simulink model "RSC_RRT_Open_Loop"  (Simulink 7.6)
settings: Solver=ode3  StartTime=0.0  StopTime=10  FixedStep=.05  RelTol=1e-3
PostLoadFcn:
  | % Setup Segmentation parameters and java class
  | % For data parsing
  | 
  | % Distance away from car to be considered
  | Threshold = 15;
  | 
  | % Maximum number of points in a clustered object
  | MaxCluster = 25;
  | 
  | % Number of data points in Lidar array
  | % DO NOT CHANGE!
  | Num_Beams = 726;
  | Scaling = 1;
  | 
  | % Get current path and import Java class
  | javaaddpath({'/'});
  | import ClusterMethodNew.*;
  | 
  | % Define instance of the class
  | DataCluster = ClusterMethodNew(Threshold,MaxCluster,Scaling);
  | 
  | % Allow reading from the workspace
  | eml.extrinsic('evalin');
InitFcn:
  | % Setup MPC parameters and Global Variables
  | a2g = 1/9.81;
  | r2d = 180/pi;
  | K_sr = 15.97;
  | neutral_steer = 104;
  | s2t = (pi/180)*(1/K_sr);
  | 
  | A_kt =[         0         0         0         0         0         0
  |          0   -3.5058   -1.6990  -25.6114   -2.2435         0
  |          0    2.2782   -4.2575  -64.1772   -5.6218         0
  |          0         0    1.0000         0         0         0
  |          0   -0.0158    0.0295    0.4442   -4.1900         0
  |          0         0         0         0    1.0000         0];
  | 
  | 
  | B_kt =[0
  |    23.7845
  |   -16.0342
  |          0
  |    17.5770
  |          0];
  | 
  | load MPC_test_2
StartFcn:
  | % Initalize serial connection with LiDAR
StopFcn:
  | % Turn off Laser and Disconnect
undefined symbols (not defined in the file or in its folder): CR, serial
libraries: instrumentlib x3, mpclib x1, realtime_pacer_lib x1
settings Model: Creator=TCA  LastModifiedBy=ipainter  BufferReuse=off
settings OptimizationCC: BlockReduction=off  InlineParams=on  BufferReuse=off  InitFltsAndDblsToZero=on
settings DebuggingCC: AlgebraicLoopMsg=none  SolverPrmCheckMsg=none  UnconnectedInputMsg=none  UnconnectedOutputMsg=none  UnconnectedLineMsg=none  StrictBusMsg=Warning
settings SFSimCC: SimParseCustomCode=off

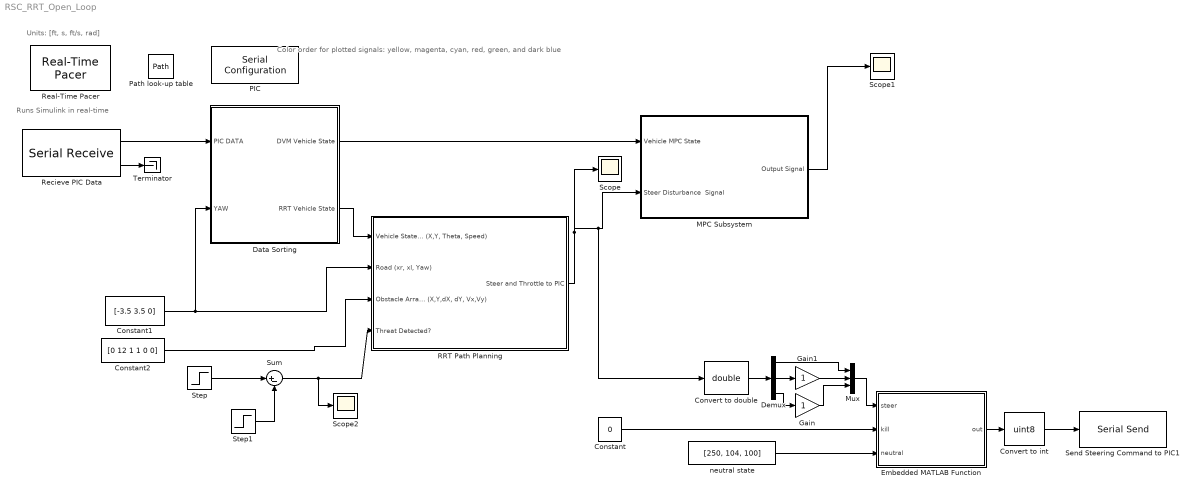
== system RSC_RRT_Open_Loop ==
  note: Runs Simulink
      |  in real-time
  note: Units: [ft, s, ft/s, rad]
  note: Color order for plotted signals:
      | yellow, magenta, cyan, red, green, and dark blue
  Constant : Constant  Value=0
  Constant1 : Constant  Value=[-3.5 3.5 0]
  Constant2 : Constant  Value=[0 12 1 1 0 0]
  Convert to double : DataTypeConversion  OutDataTypeStr=double  SampleTime=0.05  SaturateOnIntegerOverflow=on  RndMeth=Zero
  Convert to int : DataTypeConversion  OutDataTypeStr=uint8  SampleTime=0.05  SaturateOnIntegerOverflow=on  RndMeth=Zero
  Data Sorting : Subsystem
  Demux : Demux  Outputs=3
  Embedded MATLAB Function : Stateflow chart  TreatAsAtomicUnit=on
  Gain : Gain
  Gain1 : Gain
  MPC Subsystem : Subsystem
  Mux : Mux  Inputs=3
  PIC : instrumentlib/Serial Configuration  Priority=-200000  DialogController=instrumentcreatedialog  DialogControllerArgs=DataTag0  ComPortMenu=COM5  ComPort=COM5  ObjConstructor=serial('COM5');  BaudRate=9600  DataBits=8  Parity=none  StopBits=1  FlowControl=none  Timeout=10  ByteOrder=LittleEndian
  Path look-up table : DataStoreMemory  DataStoreName=Path  ReadBeforeWriteMsg=warning  WriteAfterWriteMsg=warning  WriteAfterReadMsg=warning  InitialValue=zeros(50, 6)  VectorParams1D=off
  RRT Path Planning : Subsystem
  Real-Time Pacer : realtime_pacer_lib/Real-Time Pacer  simTimePerRealTime=1
  Recieve PIC Data : instrumentlib/Serial Receive  DialogController=instrumentcreatedialog  DialogControllerArgs=DataTag1  ComPortMenu=COM5  ComPort=COM5  ObjConstructor=serial('COM5');  Terminator=CR ('\r')  DataSize="[1  16]"  DataType=uint8  EnableBlockingMode=off  ActionDataUnavailable=Output last received value  CustomValue=0  SampleTime=.05
  Scope : Scope
      settings: TimeRange=10  YMin=60  YMax=260
  Scope1 : Scope
  Scope2 : Scope
      settings: SaveName=ScopeData2
  Send Steering Command to PIC1 : instrumentlib/Serial Send  DialogController=instrumentcreatedialog  DialogControllerArgs=DataTag2  ComPortMenu=<Please select a port...>  ComPort=COM5  ObjConstructor=serial('COM5');  Header=250  Terminator=<none>  EnableBlockingMode=off
  Step : Step  Time=5  SampleTime=0
  Step1 : Step  Time=5.1  SampleTime=0
  Sum : Sum  Inputs=|+-
  Terminator : Terminator
  neutral state : Constant  Value=[250, 104, 100]
  wires:
  Data Sorting/2(RRT Vehicle State) -> RRT Path Planning/1("Vehicle State (X,Y, Theta, Speed)")
  neutral state/1 -> Embedded MATLAB Function/3(neutral)
  Embedded MATLAB Function/1(out) -> Convert to int/1
  Convert to double/1 -> Demux/1
  Demux/3 -> Gain/1
  Gain/1 -> Mux/3
  Demux/1 -> Mux/1
  Mux/1 -> Embedded MATLAB Function/1(steer)
  Demux/2 -> Gain1/1
  Gain1/1 -> Mux/2
  MPC Subsystem/1(Output Signal) -> Scope1/1
  Constant/1 -> Embedded MATLAB Function/2(kill)
  ? -> ?
  Recieve PIC Data/1 -> Data Sorting/1(PIC DATA)
  Recieve PIC Data/2 -> Terminator/1
  Constant2/1 -> RRT Path Planning/3("Obstacle Array (X,Y,dX, dY, Vx,Vy)")
  Constant1/1 -> RRT Path Planning/2("Road (xr, xl, Yaw)"), Data Sorting/2(" YAW")
  Data Sorting/1(DVM Vehicle State) -> MPC Subsystem/1(Vehicle MPC State)
  RRT Path Planning/1(Steer and Throttle to PIC) -> Scope/1, MPC Subsystem/2(Steer Disturbance  Signal), Convert to double/1
  Convert to int/1 -> Send Steering Command to PIC1/1
  Step/1 -> Sum/1
  Sum/1 -> RRT Path Planning/4(Threat Detected?), Scope2/1
  Step1/1 -> Sum/2

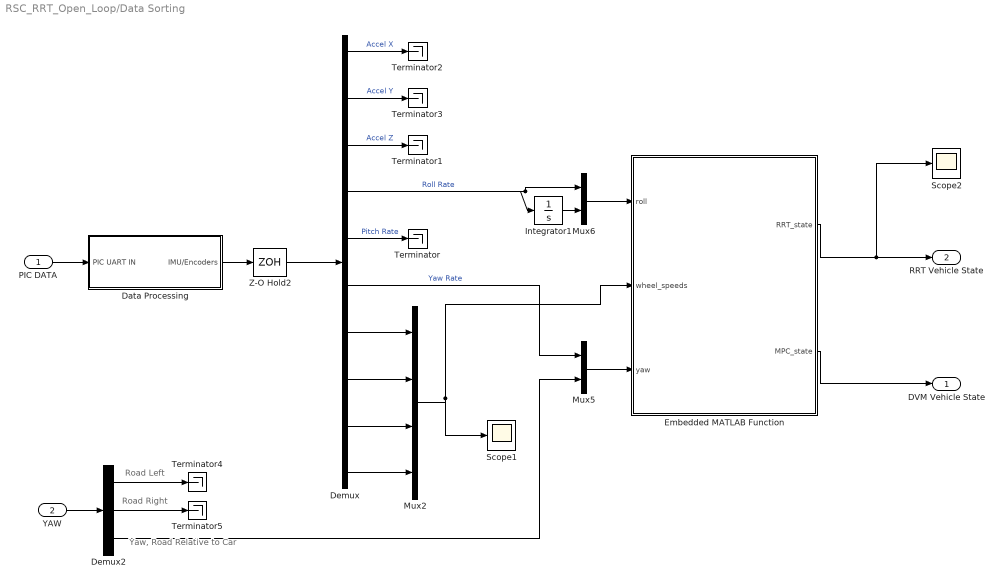
== system RSC_RRT_Open_Loop/Data Sorting ==
  note: Road Left
  note: Road Right
  note: Yaw, Road Relative to Car
  PIC DATA : Inport
  " YAW" : Inport  Port=2
  Data Processing : Subsystem
  Demux : Demux  Outputs=10
  Demux2 : Demux  Outputs=3
  Embedded MATLAB Function : Stateflow chart  TreatAsAtomicUnit=on
  Integrator1 : Integrator
  Mux2 : Mux
  Mux5 : Mux  Inputs=2
  Mux6 : Mux  Inputs=2
  Scope1 : Scope
      settings: SaveName=ScopeData3
  Scope2 : Scope
      settings: SaveName=ScopeData4
  Terminator{,1..5} (6 alike) : Terminator
  Z-O Hold2 : ZeroOrderHold  SampleTime=0.05
  DVM Vehicle State : Outport
  RRT Vehicle State : Outport  Port=2
  wires:
  Demux/6 -> Mux5/1  "Yaw Rate"
  Demux/2 -> Terminator3/1  "Accel Y"
  Demux/4 -> Mux6/1, Integrator1/1  "Roll Rate"
  Demux/5 -> Terminator/1  "Pitch Rate"
  Demux/7 -> Mux2/1
  Demux/8 -> Mux2/2
  Demux/9 -> Mux2/3
  Demux/10 -> Mux2/4
  Z-O Hold2/1 -> Demux/1
  Integrator1/1 -> Mux6/2
  Mux6/1 -> Embedded MATLAB Function/1(roll)
  Demux/1 -> Terminator2/1  "Accel X"
  Embedded MATLAB Function/2(MPC_state) -> DVM Vehicle State/1
  " YAW"/1 -> Demux2/1
  Demux/3 -> Terminator1/1  "Accel Z"
  Demux2/1 -> Terminator4/1
  Demux2/2 -> Terminator5/1
  Demux2/3 -> Mux5/2
  Mux5/1 -> Embedded MATLAB Function/3(yaw)
  Embedded MATLAB Function/1(RRT_state) -> RRT Vehicle State/1, Scope2/1
  Data Processing/1(IMU/Encoders) -> Z-O Hold2/1
  PIC DATA/1 -> Data Processing/1(PIC UART IN)
  Mux2/1 -> Embedded MATLAB Function/2(wheel_speeds), Scope1/1

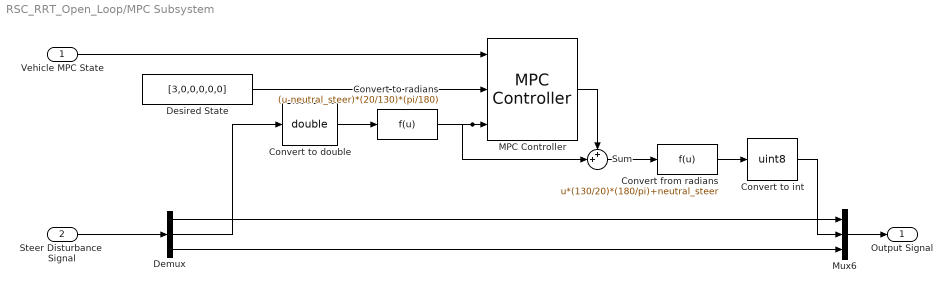
== system RSC_RRT_Open_Loop/MPC Subsystem ==
  Vehicle MPC State : Inport
  Steer Disturbance  Signal : Inport  Port=2
  Convert from radians : Fcn  Expr=u*(130/20)*(180/pi)+neutral_steer
  Convert to double : DataTypeConversion  OutDataTypeStr=double  SampleTime=.05  SaturateOnIntegerOverflow=on  RndMeth=Zero
  Convert to int : DataTypeConversion  OutDataTypeStr=uint8  SampleTime=.05  SaturateOnIntegerOverflow=on  RndMeth=Zero
  Convert to radians : Fcn  Expr=(u-neutral_steer)*(20/130)*(pi/180)
  Demux : Demux  Outputs=3
  Desired State : Constant  Value=[3,0,0,0,0,0]
  MPC Controller : mpclib/MPC Controller  SystemSampleTime=-1  mpcobj=MPC_test_2  n_mv=1  x0=[]  ref_from_ws=off  ref_signal_name=[]  ref_preview=on  md_from_ws=off  md_signal_name=[]  md_preview=on  from_project=off  md_inport=on  mv_inport=off  lims_inport=off  switch_inport=off  enable_value=0  project_file=MPCtask.mat  is_multiple=0
  Mux6 : Mux  Inputs=3
  Sum : Sum  Inputs=++|
  Output Signal : Outport
  wires:
  Convert to double/1 -> Convert to radians/1
  Desired State/1 -> MPC Controller/2
  Convert to radians/1 -> MPC Controller/3, Sum/2
  MPC Controller/1 -> Sum/1
  Steer Disturbance  Signal/1 -> Demux/1
  Demux/2 -> Convert to double/1
  Demux/1 -> Mux6/1
  Convert from radians/1 -> Convert to int/1
  Demux/3 -> Mux6/3
  Mux6/1 -> Output Signal/1
  Vehicle MPC State/1 -> MPC Controller/1
  Sum/1 -> Convert from radians/1
  Convert to int/1 -> Mux6/2

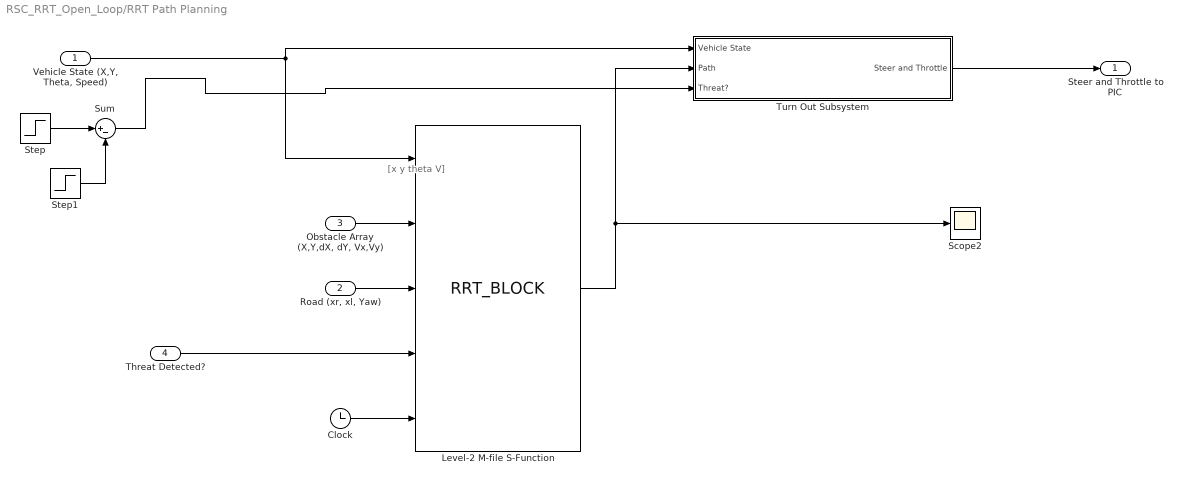
== system RSC_RRT_Open_Loop/RRT Path Planning ==
  note: [x y theta V]
  "Vehicle State (X,Y, Theta, Speed)" : Inport
  "Road (xr, xl, Yaw)" : Inport  Port=2
  "Obstacle Array (X,Y,dX, dY, Vx,Vy)" : Inport  Port=3
  Threat Detected? : Inport  Port=4
  Clock : Clock
      settings: Decimation=10
  Level-2 M-file S-Function : M-S-Function  FunctionName=RRT_BLOCK  Parameters=6
  Scope2 : Scope
      settings: SaveName=ScopeData5
  Step : Step  Time=3  SampleTime=0
  Step1 : Step  Time=7.5  SampleTime=0
  Sum : Sum  Inputs=|+-
  Turn Out Subsystem : Subsystem
  Steer and Throttle to PIC : Outport
  wires:
  Clock/1 -> Level-2 M-file S-Function/5
  "Vehicle State (X,Y, Theta, Speed)"/1 -> Level-2 M-file S-Function/1, Turn Out Subsystem/1(Vehicle State)
  "Obstacle Array (X,Y,dX, dY, Vx,Vy)"/1 -> Level-2 M-file S-Function/2
  Turn Out Subsystem/1(Steer and Throttle) -> Steer and Throttle to PIC/1
  Threat Detected?/1 -> Level-2 M-file S-Function/4
  "Road (xr, xl, Yaw)"/1 -> Level-2 M-file S-Function/3
  Step/1 -> Sum/1
  Sum/1 -> Turn Out Subsystem/3(Threat?)
  Step1/1 -> Sum/2
  Level-2 M-file S-Function/1 -> Turn Out Subsystem/2(Path), Scope2/1

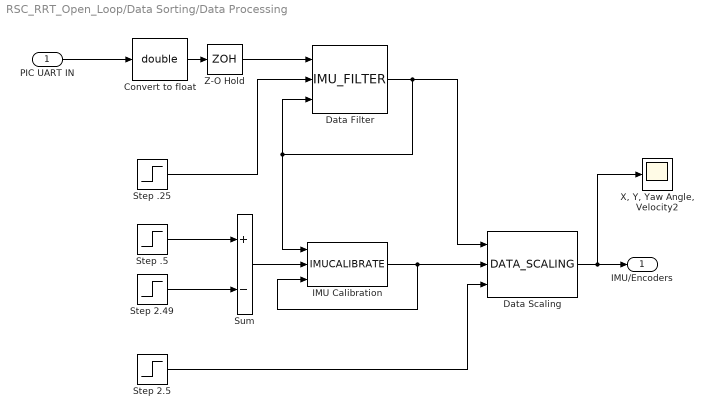
== system RSC_RRT_Open_Loop/Data Sorting/Data Processing ==
  PIC UART IN : Inport
  Convert to float : DataTypeConversion  OutDataTypeStr=double  SaturateOnIntegerOverflow=on  RndMeth=Zero
  Data Filter : M-S-Function  FunctionName=IMU_FILTER  Parameters=3
  "Data Scaling " : M-S-Function  FunctionName=DATA_SCALING  Parameters=3
  IMU Calibration : M-S-Function  FunctionName=IMUCALIBRATE  Parameters=3
  Step .25 : Step  Time=.25  SampleTime=0
  Step .5 : Step  Time=.5  SampleTime=0
  Step 2.49 : Step  Time=2.49  SampleTime=0
  Step 2.5 : Step  Time=2.5  SampleTime=0
  Sum : Sum  Inputs=+-
  "X, Y, Yaw Angle, Velocity2" : Scope
      settings: TimeRange=10  YMax=30  SaveName=ScopeData9
  Z-O Hold : ZeroOrderHold  SampleTime=0.05
  IMU/Encoders : Outport
  wires:
  Convert to float/1 -> Z-O Hold/1
  Data Filter/1 -> "Data Scaling "/1, IMU Calibration/1, Data Filter/3
  IMU Calibration/1 -> IMU Calibration/3, "Data Scaling "/2
  Step .5/1 -> Sum/1
  Step 2.49/1 -> Sum/2
  Z-O Hold/1 -> Data Filter/1
  Step .25/1 -> Data Filter/2
  Sum/1 -> IMU Calibration/2
  Step 2.5/1 -> "Data Scaling "/3
  "Data Scaling "/1 -> IMU/Encoders/1, "X, Y, Yaw Angle, Velocity2"/1
  PIC UART IN/1 -> Convert to float/1

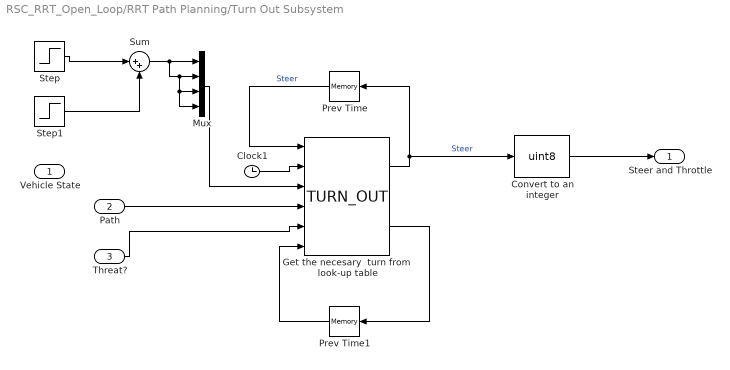
== system RSC_RRT_Open_Loop/RRT Path Planning/Turn Out Subsystem ==
  Vehicle State : Inport
  Path : Inport  Port=2
  Threat? : Inport  Port=3
  Clock1 : Clock
      settings: Decimation=10
  Convert to an integer : DataTypeConversion  OutDataTypeStr=uint8  SampleTime=.05  SaturateOnIntegerOverflow=on  RndMeth=Zero
  Get the necesary  turn from  look-up table : M-S-Function  FunctionName=TURN_OUT  Parameters=4
  Mux : Mux
  Prev Time : Memory  X0=[250 0 0]
  Prev Time1 : Memory
  Step : Step  Time=0  After=17  SampleTime=0
  Step1 : Step  Time=5  After=-5  SampleTime=0
  Sum : Sum  Inputs=|++
  Steer and Throttle : Outport
  wires:
  Get the necesary  turn from  look-up table/1 -> Prev Time/1, Convert to an integer/1  "Steer"
  Convert to an integer/1 -> Steer and Throttle/1
  Prev Time/1 -> Get the necesary  turn from  look-up table/1  "Steer"
  Get the necesary  turn from  look-up table/2 -> Prev Time1/1
  Clock1/1 -> Get the necesary  turn from  look-up table/2
  Prev Time1/1 -> Get the necesary  turn from  look-up table/6
  Threat?/1 -> Get the necesary  turn from  look-up table/5
  Path/1 -> Get the necesary  turn from  look-up table/4
  Step/1 -> Sum/1
  Step1/1 -> Sum/2
  Sum/1 -> Mux/1, Mux/2, Mux/3, Mux/4
  Mux/1 -> Get the necesary  turn from  look-up table/3

== matlab function Data Sorting/Embedded MATLAB Function ==
  data: roll input double; wheel_speeds input double; yaw input double; RRT_state output double; MPC_state output double
% Updated: May 5th, 2013

% This function takes the scaled data from the IMU and uses it to determine
% the vehicle states for the RRT and the MPC.  Note that the state of the
% vehicle is always [0 0 Yaw V]  as the coordinate system is bases on the
% postion of the vehicle.

%DATA SORTING
function [RRT_state,MPC_state]  = data_sorting(roll,wheel_speeds,yaw)

%Calculate the vehicle velocity from the wheel encoder data.  this should
%be replaced with a more robust method as this neglects the fact that the
%vechicle may be turning as well as wheel slip
velocity = (wheel_speeds(1) + wheel_speeds(2) + wheel_speeds(3) + wheel_speeds(4))/4;


Phi_d = roll(1);            % Roll Rate
Phi = roll(2);              % Roll Angle  
Psi_d = yaw(1);             % Yaw Rate
Psi = yaw(2);               % Yaw angle of the road relative to the 
                            % centerline of the car
                            
Vy = velocity;              % Velocity of the vehicle

Vx = 0;                     % Always 0 as the Coordinates are 
                            % determined by the direction of the car


MPC_state = [Vy*(1/3.28), Vx*(1/3.28), Phi_d, Phi, Psi_d, Psi]';
RRT_state = [0, 0, Psi, velocity]';

== matlab function Embedded MATLAB Function ==
  data: steer input double; kill input double; out output double; neutral input double
function out = fcn(steer,kill,neutral)
%#eml

if(kill)
    out = neutral;
else
    out = steer;
end

%end
